simulink model "Leg_4DOF_gfr_ctpid_sf"  (R2017a)
settings: Solver=FixedStepAuto  StartTime=0.0  StopTime=5  FixedStep=simulation_step  MaxStep=1e-2  RelTol=1e-3  EnableMultiTasking=on
values from neighbouring files (symbols this model uses):
  A = [ 0 ; pi/8*ones(3,1) ]    [Init_4DOF_grf_ctpid_sf.m]
  beta = 0    [Init_4DOF_grf_ctpid_sf.m]
  BodyContact = [ 4 4 ]    [Init_4DOF_grf_ctpid_sf.m]
  BodyContactPositions = [ contact_point_h, contact_point_t ]    [Init_4DOF_grf_ctpid_sf.m]
  dqInit = [ 0 0 0 0 ]'    [Init_4DOF_grf_ctpid_sf.m]
  dqInit_model = (data_steps(2,2:5)' - data_steps(1,2:5)')/(data_steps(2,1) - data_steps(1,1))    [Init_4DOF_grf_ctpid_sf.m]
  G = g*ez    [Init_4DOF_grf_ctpid_sf.m]
  G_ctrl = g*ez    [Init_4DOF_grf_ctpid_sf.m]
  h = [ ez -ey -ey -ey ]    [Init_4DOF_grf_ctpid_sf.m]
  h_ctrl = h_ctrl.*param_error    [Init_4DOF_grf_ctpid_sf.m]
  Inertia = [ I_base I_hip I_thigh I_shin I_foot ]    [Init_4DOF_grf_ctpid_sf.m]
  Inertia_ctrl = Inertia_ctrl.*param_error    [Init_4DOF_grf_ctpid_sf.m]
  joint_type = [ 1 0 0 0 ]    [Init_4DOF_grf_ctpid_sf.m]
  k_b = 50000    [Init_4DOF_grf_ctpid_sf.m]
  k_noise = 0    [Init_4DOF_grf_ctpid_sf.m]
  Kd = kd*eye(n)    [Init_4DOF_grf_ctpid_sf.m]
  Ki = ki*eye(n)    [Init_4DOF_grf_ctpid_sf.m]
  Kp = kp*eye(n)    [Init_4DOF_grf_ctpid_sf.m]
  L = [ l_base_hip l_hip_thigh l_thigh_shin l_shin_foot ]    [Init_4DOF_grf_ctpid_sf.m]
  L_ctrl = L_ctrl.*param_error    [Init_4DOF_grf_ctpid_sf.m]
  Mass = [ mass_base mass_hip mass_thigh mass_shin mass_foot ]    [Init_4DOF_grf_ctpid_sf.m]
  Mass_ctrl = Mass_ctrl.*param_error    [Init_4DOF_grf_ctpid_sf.m]
  n = 4    [Init_4DOF_grf_ctpid_sf.m]
  offset = zeros(n,1)    [Init_4DOF_grf_ctpid_sf.m]
  qInit = [ 0.0216 0.5675 -0.13 -0.39 ]'    [Init_4DOF_grf_ctpid_sf.m]
  qInit_model = qInit    [Init_4DOF_grf_ctpid_sf.m]
  R = [ r_base r_hip r_thigh r_shin r_foot ]    [Init_4DOF_grf_ctpid_sf.m]
  R_ctrl = R_ctrl.*param_error    [Init_4DOF_grf_ctpid_sf.m]
  s_z = 1    [Init_4DOF_grf_ctpid_sf.m]
  simulation_step = 1e-4    (= 0.0001)    [Init_4DOF_grf_ctpid_sf.m]
  tau = 0.001    [Init_4DOF_grf_ctpid_sf.m]
  w = [ 0   ; 2*pi/2*ones(3,1) ]    [Init_4DOF_grf_ctpid_sf.m]
  wn_ref = 8*5    (= 40)    [Init_4DOF_grf_ctpid_sf.m]
  zeta_ref = 0.7    [Init_4DOF_grf_ctpid_sf.m]
libraries: simulink x1
settings Model: Creator=Ultron  LastModifiedBy=igricart
settings DataIOCC: LimitDataPoints=on  SaveFormat=Array
settings OptimizationCC: LifeSpan=inf
settings DebuggingCC: SFUnexpectedBacktrackingDiag=warning  SFNoUnconditionalDefaultTransitionDiag=warning  SFExecutionAtInitializationDiag=none
settings HardwareCC: ProdBitPerPointer=32  ProdBitPerSizeT=32  ProdBitPerPtrDiffT=32  ProdLargestAtomicFloat=None  ProdIntDivRoundTo=Undefined  ProdEndianess=Unspecified  ProdWordSize=32  ProdHWDeviceType=32-bit Generic
settings ModelReferenceCC: PropagateSignalLabelsOutOfModel=off
settings GRTTargetCC: TargetLangStandard=C89/C90 (ANSI)  GeneratePreprocessorConditionals=Disable all
settings ConfigComp: CovMetricSettings=dw  CovHtmlReporting=on  CovSaveCumulativeToWorkspaceVar=on  CovSaveSingleToWorkspaceVar=on  CovExternalEMLEnable=off

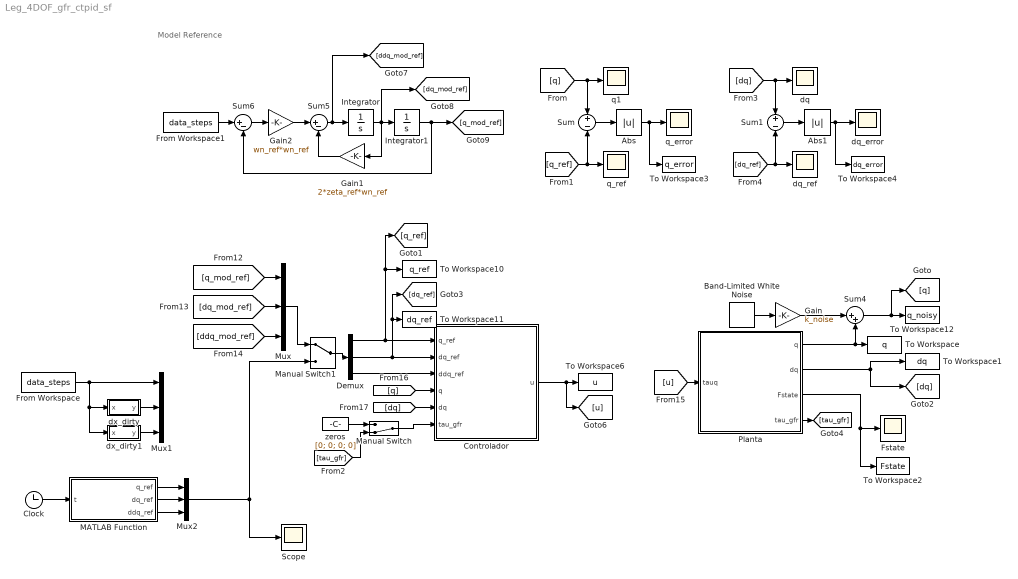
== system Leg_4DOF_gfr_ctpid_sf ==
  note: Model Reference
  Abs : Abs
  Abs1 : Abs
  Band-Limited White Noise : simulink/Sources/Band-Limited White Noise  Cov=[0.1]  Ts=simulation_step  seed=[23341]
  Clock : Clock
  Controlador : Subsystem
  Demux : Demux  Outputs=3
  From Workspace : FromWorkspace  VariableName=data_steps  SampleTime=0
  From Workspace1 : FromWorkspace  VariableName=data_steps  SampleTime=0
  Fstate : Scope
  Gain : Gain  Gain=k_noise
  Gain1 : Gain  Gain=2*zeta_ref*wn_ref
  Gain2 : Gain  Gain=wn_ref*wn_ref
  Integrator : Integrator  InitialCondition=dqInit_model
  Integrator1 : Integrator  InitialCondition=qInit_model
  MATLAB Function : MATLAB Function  TreatAsAtomicUnit=on
  Manual Switch : ManualSwitch  CurrentSetting=0
  Manual Switch1 : ManualSwitch
  Mux : Mux  Inputs=3
  Mux1 : Mux  Inputs=3
  Mux2 : Mux  Inputs=3
  Planta : Subsystem
  Scope : Scope
  Sum : Sum  Inputs=+-
  Sum1 : Sum  Inputs=+-
  Sum4 : Sum  Inputs=|++
  Sum5 : Sum  Inputs=|+-
  Sum6 : Sum  Inputs=|+-
  To Workspace : ToWorkspace  VariableName=q  SaveFormat=Timeseries  SampleTime=-1
  To Workspace1 : ToWorkspace  VariableName=dq  SaveFormat=Timeseries  SampleTime=-1
  To Workspace10 : ToWorkspace  VariableName=q_ref  SaveFormat=Timeseries  SampleTime=-1
  To Workspace11 : ToWorkspace  VariableName=dq_ref  SaveFormat=Timeseries  SampleTime=-1
  To Workspace12 : ToWorkspace  VariableName=q_noisy  SaveFormat=Timeseries  SampleTime=-1
  To Workspace2 : ToWorkspace  VariableName=Fstate  SaveFormat=Timeseries  SampleTime=-1
  To Workspace3 : ToWorkspace  VariableName=q_error  SaveFormat=Timeseries  SampleTime=-1
  To Workspace4 : ToWorkspace  VariableName=dq_error  SaveFormat=Timeseries  SampleTime=-1
  To Workspace6 : ToWorkspace  VariableName=u  SaveFormat=Timeseries  SampleTime=-1
  dq : Scope
  dq_error : Scope
  dq_ref : Scope
  dx_dirty : Subsystem
  dx_dirty1 : Subsystem
  q1 : Scope
  q_error : Scope
  q_ref : Scope
  zeros : Constant  Value=[0; 0; 0; 0]
  wires:
  [q] -> q1/1, Sum/1
  [q_ref] -> q_ref/1, Sum/2
  Sum/1 -> Abs/1
  Abs/1 -> To Workspace3/1, q_error/1
  [dq_ref] -> dq_ref/1, Sum1/2
  Sum1/1 -> Abs1/1
  Abs1/1 -> To Workspace4/1, dq_error/1
  [dq] -> dq/1, Sum1/1
  Sum4/1 -> [q], To Workspace12/1
  Band-Limited White Noise/1 -> Gain/1
  Planta/1(q) -> Sum4/2, To Workspace/1
  Planta/3(Fstate) -> To Workspace2/1, Fstate/1
  Planta/2(dq) -> To Workspace1/1, [dq]
  Gain/1 -> Sum4/1
  [u] -> Planta/1(tauq)
  Demux/2 -> Controlador/2(dq_ref), To Workspace11/1, [dq_ref]
  [q] -> Controlador/4(q)
  Demux/1 -> To Workspace10/1, [q_ref], Controlador/1(q_ref)
  From Workspace/1 -> Mux1/1, dx_dirty1/1(x), dx_dirty/1(x)
  Manual Switch1/1 -> Demux/1
  [dq_mod_ref] -> Mux/2
  [q_mod_ref] -> Mux/1
  dx_dirty/1(y) -> Mux1/2
  [ddq_mod_ref] -> Mux/3
  dx_dirty1/1(y) -> Mux1/3
  Mux/1 -> Manual Switch1/1
  [dq] -> Controlador/5(dq)
  Demux/3 -> Controlador/3(ddq_ref)
  Controlador/1(u) -> [u], To Workspace6/1
  From Workspace1/1 -> Sum6/1
  Gain2/1 -> Sum5/1
  Gain1/1 -> Sum5/2
  Sum6/1 -> Gain2/1
  Sum5/1 -> Integrator/1, [ddq_mod_ref]
  Integrator/1 -> [dq_mod_ref], Gain1/1, Integrator1/1
  Integrator1/1 -> [q_mod_ref], Sum6/2
  Planta/4(tau_gfr) -> [tau_gfr]
  Manual Switch/1 -> Controlador/6(tau_gfr)
  [tau_gfr] -> Manual Switch/2
  zeros/1 -> Manual Switch/1
  Clock/1 -> MATLAB Function/1(t)
  MATLAB Function/1(q_ref) -> Mux2/1
  MATLAB Function/2(dq_ref) -> Mux2/2
  MATLAB Function/3(ddq_ref) -> Mux2/3
  Mux2/1 -> Scope/1, Manual Switch1/2

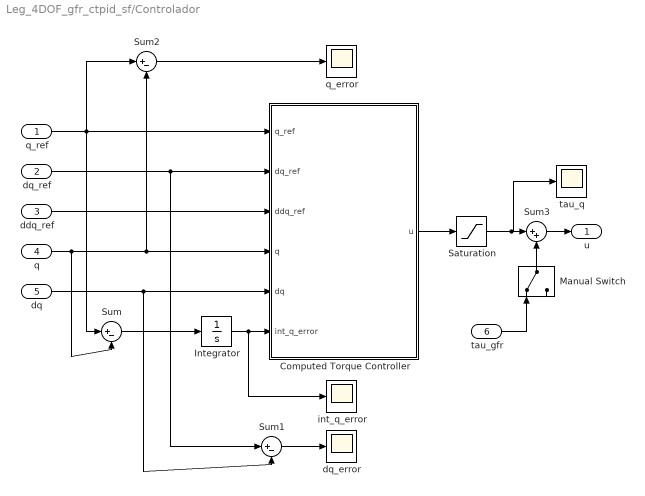
== system Leg_4DOF_gfr_ctpid_sf/Controlador ==
  q_ref : Inport
  dq_ref : Inport  Port=2
  ddq_ref : Inport  Port=3
  q : Inport  Port=4
  dq : Inport  Port=5
  tau_gfr : Inport  Port=6
  Computed Torque Controller : MATLAB Function  TreatAsAtomicUnit=on
  Integrator : Integrator  InitialCondition=zeros(4,1)
  Manual Switch : ManualSwitch
  Saturation : Saturate  UpperLimit=800  LowerLimit=-800
  Sum : Sum  Inputs=|+-
  Sum1 : Sum  Inputs=|+-
  Sum2 : Sum  Inputs=|+-
  Sum3 : Sum  Inputs=|++
  dq_error : Scope
  int_q_error : Scope
  q_error : Scope
  tau_q : Scope
  u : Outport
  wires:
  Computed Torque Controller/1(u) -> Saturation/1
  q_ref/1 -> Sum2/1, Sum/1, Computed Torque Controller/1(q_ref)
  dq_ref/1 -> Sum1/1, Computed Torque Controller/2(dq_ref)
  q/1 -> Sum/2, Computed Torque Controller/4(q), Sum2/2
  Sum1/1 -> dq_error/1
  ddq_ref/1 -> Computed Torque Controller/3(ddq_ref)
  dq/1 -> Sum1/2, Computed Torque Controller/5(dq)
  Sum/1 -> Integrator/1
  Integrator/1 -> int_q_error/1, Computed Torque Controller/6(int_q_error)
  Sum2/1 -> q_error/1
  Saturation/1 -> Sum3/1, tau_q/1
  Sum3/1 -> u/1
  Manual Switch/1 -> Sum3/2
  tau_gfr/1 -> Manual Switch/1

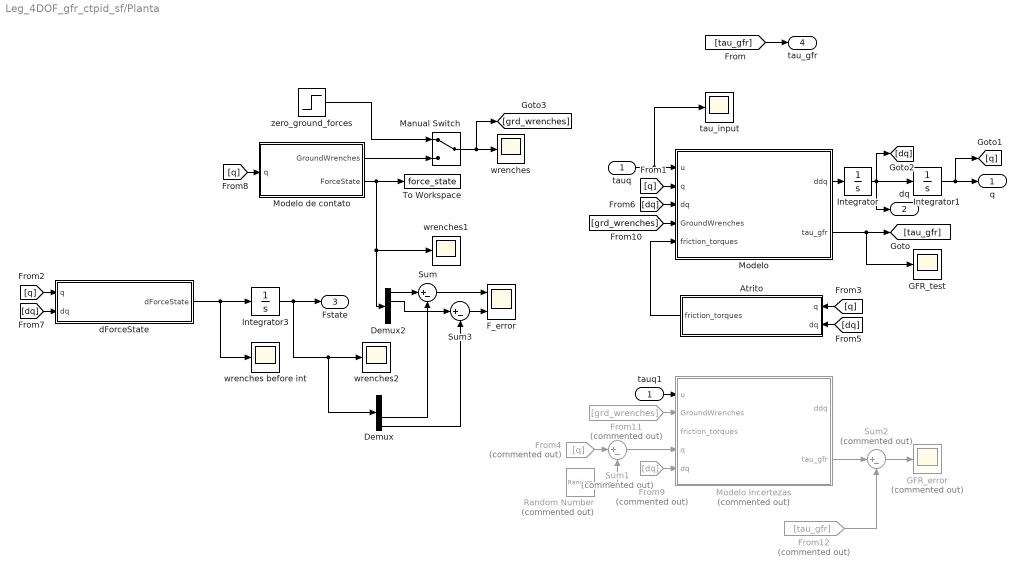
== system Leg_4DOF_gfr_ctpid_sf/Planta ==
  tauq : Inport
  Atrito : MATLAB Function  TreatAsAtomicUnit=on
  Demux : Demux
  Demux2 : Demux
  F_error : Scope  NumInputPorts=2
  From11 : From  Commented=on  GotoTag=grd_wrenches
  From12 : From  Commented=on  GotoTag=tau_gfr
  From4 : From  Commented=on  GotoTag=q
  From9 : From  Commented=on  GotoTag=dq
  GFR_error : Scope  Commented=on
  GFR_test : Scope
  Integrator : Integrator  InitialCondition=dqInit
  Integrator1 : Integrator  InitialCondition=qInit
  Integrator3 : Integrator  InitialCondition=zeros(1,4)
  Manual Switch : ManualSwitch
  Modelo : MATLAB Function  TreatAsAtomicUnit=on
  Modelo Incertezas : MATLAB Function  Commented=on  TreatAsAtomicUnit=on
  Modelo de contato : MATLAB Function  TreatAsAtomicUnit=on
  Random Number : RandomNumber  Commented=on  Variance=2*pi/(360*1e6)  SampleTime=simulation_step
  Sum : Sum  Inputs=|+-
  Sum1 : Sum  Commented=on  Inputs=|+-
  Sum2 : Sum  Commented=on  Inputs=|+-
  Sum3 : Sum  Inputs=|+-
  To Workspace : ToWorkspace  VariableName=force_state  SaveFormat=Timeseries  SampleTime=-1
  dForceState : MATLAB Function  TreatAsAtomicUnit=on
  tau_input : Scope
  tauq1 : InportShadow
  wrenches : Scope
  wrenches before int : Scope
  wrenches1 : Scope
  wrenches2 : Scope
  zero_ground_forces : Step  Before=zeros(6,2)  After=zeros(6,2)  SampleTime=0
  q : Outport
  dq : Outport  Port=2
  Fstate : Outport  Port=3
  tau_gfr : Outport  Port=4
  wires:
  Integrator1/1 -> [q], q/1
  Integrator/1 -> dq/1, [dq], Integrator1/1
  Atrito/1(friction_torques) -> Modelo/5(friction_torques)
  Integrator3/1 -> Demux/1, wrenches2/1, Fstate/1
  Modelo de contato/2(ForceState) -> To Workspace/1, wrenches1/1, Demux2/1
  Manual Switch/1 -> [grd_wrenches], wrenches/1
  Modelo de contato/1(GroundWrenches) -> Manual Switch/2
  zero_ground_forces/1 -> Manual Switch/1
  Modelo/1(ddq) -> Integrator/1
  Modelo/2(tau_gfr) -> GFR_test/1, [tau_gfr]
  tauq/1 -> tau_input/1, Modelo/1(u)
  [tau_gfr] -> tau_gfr/1
  tauq1/1 -> Modelo Incertezas/1(u)
  [q] -> Modelo/2(q)
  [q] -> dForceState/1(q)
  [q] -> Atrito/1(q)
  [dq] -> Atrito/2(dq)
  [dq] -> Modelo/3(dq)
  [dq] -> dForceState/2(dq)
  [q] -> Modelo de contato/1(q)
  From9/1 -> Modelo Incertezas/5(dq)
  [grd_wrenches] -> Modelo/4(GroundWrenches)
  From11/1 -> Modelo Incertezas/2(GroundWrenches)
  Sum1/1 -> Modelo Incertezas/4(q)
  From4/1 -> Sum1/1
  Random Number/1 -> Sum1/2
  Modelo Incertezas/2(tau_gfr) -> Sum2/1
  From12/1 -> Sum2/2
  Sum2/1 -> GFR_error/1
  dForceState/1(dForceState) -> wrenches before int/1, Integrator3/1
  Demux2/1 -> Sum/1
  Demux/3 -> Sum/2
  Demux/4 -> Sum3/2
  Sum3/1 -> F_error/2
  Sum/1 -> F_error/1
  Demux2/2 -> Sum3/1

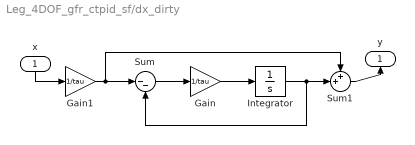
== system Leg_4DOF_gfr_ctpid_sf/dx_dirty ==
  x : Inport
  Gain : Gain  Gain=1/tau
  Gain1 : Gain  Gain=1/tau
  Integrator : Integrator  InitialCondition=dqInit
  Sum : Sum  Inputs=|--
  Sum1 : Sum  Inputs=++|
  y : Outport
  wires:
  Gain1/1 -> Sum1/1, Sum/1
  x/1 -> Gain1/1
  Gain/1 -> Integrator/1
  Integrator/1 -> Sum/2, Sum1/2
  Sum/1 -> Gain/1
  Sum1/1 -> y/1

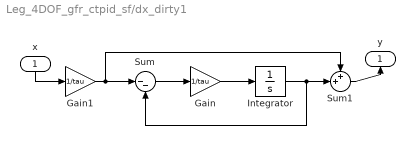
== system Leg_4DOF_gfr_ctpid_sf/dx_dirty1 ==
  x : Inport
  Gain : Gain  Gain=1/tau
  Gain1 : Gain  Gain=1/tau
  Integrator : Integrator  InitialCondition=zeros(4,1)
  Sum : Sum  Inputs=|--
  Sum1 : Sum  Inputs=++|
  y : Outport
  wires:
  Sum1/1 -> y/1
  Sum/1 -> Gain/1
  Integrator/1 -> Sum1/2, Sum/2
  Gain/1 -> Integrator/1
  x/1 -> Gain1/1
  Gain1/1 -> Sum/1, Sum1/1

== matlab function Leg_4DOF_gfr_ctpid_sf/Controlador/Computed Torque Controller ==
  data: q_ref input; dq_ref input; ddq_ref input; u output; q input; dq input; int_q_error input; joint_type parameter; Mass_ctrl parameter; Inertia_ctrl parameter; R_ctrl parameter; L_ctrl parameter; h_ctrl parameter; G_ctrl parameter; Kp parameter; Kd parameter; Ki parameter
function u = fcn(q_ref, dq_ref, ddq_ref, q, dq, int_q_error, joint_type, Mass_ctrl, Inertia_ctrl, R_ctrl, L_ctrl, h_ctrl, G_ctrl, Kp, Kd, Ki )
%% Prostectics control

v = ddq_ref + Kd*(dq_ref - dq) + Kp*(q_ref - q) + Ki*int_q_error;
u = prosthetics_inverse_dynamics( q, dq, v, joint_type, Mass_ctrl, Inertia_ctrl, R_ctrl, L_ctrl, h_ctrl, G_ctrl );

== matlab function Leg_4DOF_gfr_ctpid_sf/Planta/Modelo ==
  data: u input; q input; dq input; GroundWrenches input; friction_torques input; joint_type parameter; Mass parameter; Inertia parameter; R parameter; L parameter; h parameter; G parameter; ddq output; BodyContactPositions parameter; BodyContact parameter; tau_gfr output
function [ddq, tau_gfr] = fcn( u, q, dq, GroundWrenches, friction_torques, joint_type, Mass, Inertia, R, L, h, G, BodyContactPositions,  BodyContact )
% direct dynamics

% n = length(q);

% coder.extrinsic('model_prosthetics_mex');
% ddq = coder.nullcopy(zeros(n,1));
% Friction_torques = coder.nullcopy(zeros(n,1));

[ddq, tau_gfr] = model_prosthetics( u, q, dq, joint_type, Mass, Inertia, R, L, h, G, friction_torques, BodyContact, GroundWrenches, BodyContactPositions );
% ddq = model_prosthetics_mex( u, q, dq, joint_type, Mass, Inertia, R, L, h, G, friction_coefs, BodyContact, BodyContactWrenches, BodyContactPositions );

== matlab function Leg_4DOF_gfr_ctpid_sf/Planta/Modelo Incertezas ==
  data: u input; GroundWrenches input; friction_torques input; q input; dq input; joint_type parameter; Mass parameter; Inertia parameter; R parameter; L parameter; h parameter; G parameter; ddq output; BodyContactPositions parameter; BodyContact parameter; tau_gfr output
function [ddq, tau_gfr] = fcn( u, GroundWrenches, friction_torques, q, dq, joint_type, Mass, Inertia, R, L, h, G, BodyContactPositions,  BodyContact )
% direct dynamics

% n = length(q);

% coder.extrinsic('model_prosthetics_mex');
% ddq = coder.nullcopy(zeros(n,1));
% Friction_torques = coder.nullcopy(zeros(n,1));

[ddq, tau_gfr] = model_prosthetics( u, q, dq, joint_type, Mass, Inertia, R, L, h, G, friction_torques, BodyContact, GroundWrenches, BodyContactPositions );
% ddq = model_prosthetics_mex( u, q, dq, joint_type, Mass, Inertia, R, L, h, G, friction_coefs, BodyContact, BodyContactWrenches, BodyContactPositions );

== matlab function Leg_4DOF_gfr_ctpid_sf/Planta/Atrito ==
  data: friction_torques output; q input; dq input
function friction_torques = fcn( q, dq )
%% Joint friction model
n = length(q);
friction_torques = zeros(n,1);

== matlab function Leg_4DOF_gfr_ctpid_sf/MATLAB Function ==
  data: t input; q_ref output; dq_ref output; ddq_ref output; n parameter; A parameter; offset parameter; w parameter
function [ q_ref, dq_ref, ddq_ref ] = fcn( t, n,  A, offset, w)
% generate reference

q_ref = A.*sin(w.*t + offset);
dq_ref = A.*w.*cos(w.*t + offset);
ddq_ref = -A.*(w.^2).*sin(w.*t + offset);

% q_ref = zeros(n,1);
% dq_ref = zeros(n,1);
% ddq_ref = zeros(n,1);
% 
% for i = 1:n
%     q_ref(i) = A(i)*sin(w(i)*t + offset(i));
%     dq_ref(i) = A(i)*w(i)*cos(w(i)*t + offset(i));
%     ddq_ref(i) = -A(i)*(w(i)^2)*sin(w(i)*t + offset(i));
% end

== matlab function Leg_4DOF_gfr_ctpid_sf/Planta/Modelo de contato ==
  data: GroundWrenches output; q input; BodyContactPositions parameter; s_z parameter; L parameter; h parameter; beta parameter; k_b parameter; joint_type parameter; ForceState output
function [ GroundWrenches, ForceState ] = fcn( q, BodyContactPositions, s_z, L, h, beta,  k_b, joint_type )
% function BodyContactWrenches = fcn( t, q, L, h, BodyContactPositions, joint_type, sz, beta, kb)
% Esta função calcula as forças de contato com o chão

[ GroundWrenches, ForceState ] = ground_model( q, BodyContactPositions, s_z, L, h, beta,  k_b, joint_type );

== matlab function Leg_4DOF_gfr_ctpid_sf/Planta/dForceState ==
  data: q input; dq input; dForceState output; L parameter; h parameter; joint_type parameter; BodyContactPositions parameter; s_z parameter; beta parameter; k_b parameter
function dForceState = fcn( q, dq, L, h, joint_type,  BodyContactPositions, s_z, beta, k_b)
%% Dinâmica do modelo de contato (em coordenadas inerciais)

%% Computes the velocity body twist of the given point.
body = 4;
contact_point_h = BodyContactPositions(:,1);
contact_point_t = BodyContactPositions(:,2);
V_h = prosthetics_diff_kinematics( q, dq, L, h, body, contact_point_h, joint_type );
V_t = prosthetics_diff_kinematics( q, dq, L, h, body, contact_point_t, joint_type );

%% Computes 
[ P_h, R_h ] = prosthetics_forward_kinematics( q, L, h, body, contact_point_h, joint_type );
[ P_t, R_t ] = prosthetics_forward_kinematics( q, L, h, body, contact_point_t, joint_type );
z_h = P_h(3);
z_t = P_t(3);

%% Leg parameters according to Fakoorian paper
l2 = L(3,3);
l3 = L(3,4);
ah = contact_point_h(3);
aH = norm(contact_point_h);
aT = norm(contact_point_t);

%% Converts body linear velocity into inertial velocty
v_h = R_h*V_h(1:3);
v_t = R_t*V_t(1:3);

% Recursive Solution
dz_h = v_h(3);
dz_t = v_t(3);

dF_zh = -(k_b/2)*dz_h*(1+sign(z_h - s_z));
dF_zt = -(k_b/2)*dz_t*(1+sign(z_t - s_z));

dF_xh = beta*dF_zh;
dF_xt = beta*dF_zt;

% Analitical solution
anal_z_h = q(1) + l2 * cos( q(2) ) + l3 * ( cos( q(2) + q(3) ) ) ...
    + aH * cos( q(2) + q(3) + q(4) + ( - acos( ah / aH ) ) );

anal_z_t = q(1) + l2 * cos( q(2) ) + l3 * ( cos( q(2) + q(3) ) ) ...
    + aT * cos( q(2) + q(3) + q(4) + ( acos( ah / aT ) ) );

anal_dz_h = dq(1) - dq(2) * l2 * sin( q(2) ) - ( dq(2) + dq(3) ) * l3 * ( sin( q(2) + q(3) ) ) ...
    - ( dq(2) + dq(3) + dq(4) ) * aH * sin( q(2) + q(3) + q(4) + ( - acos( ah / aH ) ) );

anal_dz_t = dq(1) - dq(2) * l2 * sin( q(2) ) - ( dq(2) + dq(3) ) * l3 * ( sin( q(2) + q(3) ) ) ...
    - ( dq(2) + dq(3) + dq(4) ) * aT * sin( q(2) + q(3) + q(4) + ( acos( ah / aT ) ) );

anal_dF_zh = -(k_b/2)*anal_dz_h*(1+sign(z_h - s_z));
anal_dF_zt = -(k_b/2)*anal_dz_t*(1+sign(z_t - s_z));

erro_zh = anal_z_h - z_h;
erro_zt = anal_z_t - z_t; 

dForceState = [ dF_zh, dF_zt, anal_dF_zh, anal_dF_zt]';
